simulink model "seminar4_topic1"  (R2019b)
settings: Solver=VariableStepAuto  StartTime=0.0  StopTime=0.2  RelTol=1e-3
model workspace (MAT data in the model file):
  d = 25
libraries: powerlib x10
settings Model: ParameterArgumentNames=d  OrderedModelArguments=off  Creator=Lenovo  LastModifiedBy=96547
settings DataIOCC: ReturnWorkspaceOutputs=off

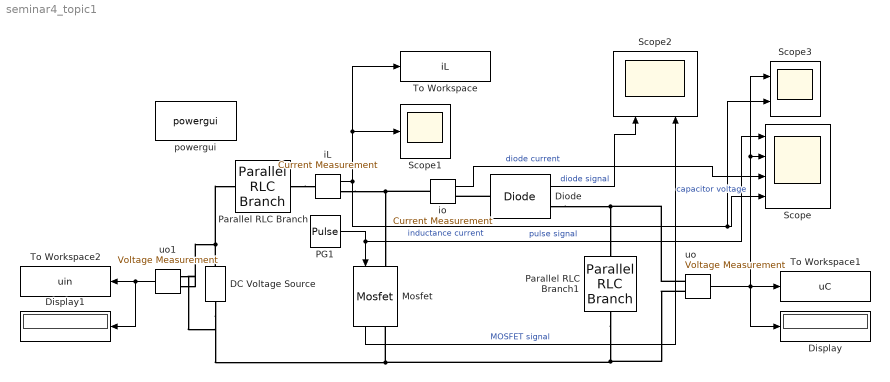
== system seminar4_topic1 ==
  DC Voltage Source : powerlib/Electrical Sources/DC Voltage Source  Amplitude=300  Measurements=None
  Diode : powerlib/Power Electronics/Diode  Ron=0.001  Lon=0  Vf=0.8  IC=0  UseSnubber=0  Rs=500  Cs=250e-9  Measurements=on
  Display : Display
  Display1 : Display
  Mosfet : powerlib/Power Electronics/Mosfet  Ron=0.1  Lon=0  Rd=0.01  Vfd=0  IC=0  Rs=1e5  Cs=inf  Measurements=on
  PG1 : DiscretePulseGenerator  PulseType=Time based  Period=1e-5  PulseWidth=25
  Parallel RLC Branch : powerlib/Elements/Parallel RLC Branch  LConnTagsString=a  RConnTagsString=__new0  BranchType=L  Resistance=1  Inductance=800e-6  SetiL0=off  InitialCurrent=0  Capacitance=1e-6  Setx0=off  InitialVoltage=0  Measurements=None
  Parallel RLC Branch1 : powerlib/Elements/Parallel RLC Branch  LConnTagsString=a  RConnTagsString=__new0  BranchType=RC  Resistance=100  Inductance=1e-3  SetiL0=off  InitialCurrent=0  Capacitance=200e-6  Setx0=off  InitialVoltage=0  Measurements=Branch voltage and current
  Scope : Scope  NumInputPorts=4
  Scope1 : Scope
  Scope2 : Scope  NumInputPorts=2
  Scope3 : Scope  NumInputPorts=2
  To Workspace : ToWorkspace  VariableName=iL  SampleTime=-1
      settings: Save2DSignal=2-D array (concatenate along first dimension)
  To Workspace1 : ToWorkspace  VariableName=uC  SampleTime=-1
      settings: Save2DSignal=2-D array (concatenate along first dimension)
  To Workspace2 : ToWorkspace  VariableName=uin  SampleTime=-1
      settings: Save2DSignal=2-D array (concatenate along first dimension)
  iL : powerlib/Measurements/Current Measurement  PhasorSimulation=off  OutputType=Complex  PSBequivalent=0
  io : powerlib/Measurements/Current Measurement  PhasorSimulation=off  OutputType=Complex  PSBequivalent=0
  powergui : powerlib/powergui  Priority=1  SimulationMode=Continuous  SampleTime=50e-6  frequency=60  Iterations=50  frequencyindice=0  Pbase=100e6  ErrMax=1e-4  UnitsV=kV  UnitsW=MW  buscounter=0  FunctionMessages=off  echomessages=off  EnableUseOfTLC=off  CurrentSourceSwitches=off  DisableSnubberDevices=off  DisableRonSwitches=off  DisableVfSwitches=off  DisplayEquations=off  AutomaticDiscreteSolvers=off  SolverType=Tustin/Backward Euler (TBE)  Interpol=off  ExternalGateDelay=off  methode=off  Ts=100  x0status=blocks  SPID=on  SwTol=0  HookPort=off  NonlinearTolerance=1e-4  nMaxIteration=100  ContinueOnMaxIteration=off  RestoreLinks=warning  ResistiveCurrentMeasurement=off  Frange=[0:2:500]  Ylog=off  Xlog=on  ShowGrid=off  save=off  variable=ZData  structure=0  ZoomFFT=off  StartTime=0.0  cycles=1  DisplayStyle=1  fundamental=60  FreqAxis=off  MaxFrequency=1000  frequencyindicesteady=1  RmsSteady=1  display=off
      settings: SourceProductName=Simscape Electrical
  uo : powerlib/Measurements/Voltage Measurement  PhasorSimulation=off  OutputType=Complex  PSBequivalent=0
  uo1 : powerlib/Measurements/Voltage Measurement  PhasorSimulation=off  OutputType=Complex  PSBequivalent=0
  wires:
  io/1 -> Scope/3  "diode current"
  uo/1 -> Scope3/1, Scope/2, Display/1, To Workspace1/1  "capacitor voltage"
  PG1/1 -> Mosfet/1, Scope/1  "pulse signal"
  iL/1 -> Scope3/2, Scope/4, To Workspace/1, Scope1/1  "inductance current"
  Diode/1 -> Scope2/1  "diode signal"
  Mosfet/1 -> Scope2/2  "MOSFET signal"
  uo1/1 -> Display1/1, To Workspace2/1
  connections:
  DC Voltage Source/RConn1 -- uo1/LConn1 -- Parallel RLC Branch/LConn1
  io/LConn1 -- iL/RConn1 -- Mosfet/LConn1
  Diode/LConn1 -- io/RConn1
  Diode/RConn1 -- Parallel RLC Branch1/LConn1 -- uo/LConn1
  Parallel RLC Branch1/RConn1 -- uo/LConn2 -- uo1/LConn2 -- DC Voltage Source/LConn1 -- Mosfet/RConn1
  Parallel RLC Branch/RConn1 -- iL/LConn1
